simulink model "self_play"  (R2013b)
settings: Solver=ode45  StartTime=0.0  StopTime=3  RelTol=1e-3
libraries: dspsigops x1
settings Model: Creator=yz10g11  LastModifiedBy=yz10g11

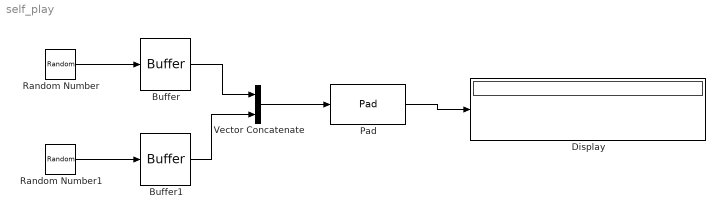
== system self_play ==
  Buffer : Buffer  N=3  TreatMby1Signals=One channel
  Buffer1 : Buffer  N=3  TreatMby1Signals=One channel
  Display : Display
  Pad : dspsigops/Pad  padAlong=Rows  dimsToPad=1  valSrc=Specify via dialog  padVal=0  spec=Output size  padNumOutRowsSpecMethod=User-specified  numOutRows=1  padNumOutColsSpecMethod=User-specified  numOutCols=3  isVarDimsMode=off  padBeginning=0  padEnd=0  outSizeMode=User-specified  outSize=1  padSigAt=End  trunc_flag=None  roundingMode=Floor  overflowMode=off  truncOrWrapMode=Truncate  wrap_flag=None
  Random Number : RandomNumber  SampleTime=1
  Random Number1 : RandomNumber  SampleTime=1
  Vector Concatenate : Concatenate  Mode=Multidimensional array  ConcatenateDimension=2
  wires:
  Random Number/1 -> Buffer/1
  Random Number1/1 -> Buffer1/1
  Buffer/1 -> Vector Concatenate/1
  Buffer1/1 -> Vector Concatenate/2
  Vector Concatenate/1 -> Pad/1
  Pad/1 -> Display/1
